simulink model "pid_controller_4inj_dll"  (Simulink 4.00)
settings: Solver=ode5  SolverMode=SingleTasking  StartTime=0.0  StopTime=10  FixedStep=0.0005  RelTol=1e-3
settings Model: Creator=mandic  LastModifiedBy=CAIKA  ExternalInput=[u]  RTWOptions="-aEnforceIntegerDowncast=1 -aExtMode=0 -aFoldNonRolledExpr=1 -aForceParamTrailComments=0 -aGenerateComments=1 -aIgnoreCustomStorageClasses=0 -aIncHierarchyInIds=0 -aInlineInvariantSignals=0 -aLocalBlockOutputs=1 -aLogVarNameModifier=\"rt_\" -aRTWVerbose=1 -aRollThreshold=5 -aShowEliminatedStatements=1"  RTWRetainRTWFile=on  RTWTemplateMakefile=avl_grt_dll_nt.tmf  RTWMakeCommand=make_rtw PROGRAM=pid_controller_4inj  ExtModeTrigMode=oneshot  ExtModeArmWhenConnect=off  ExtModeAutoUpdateStatusClock=off

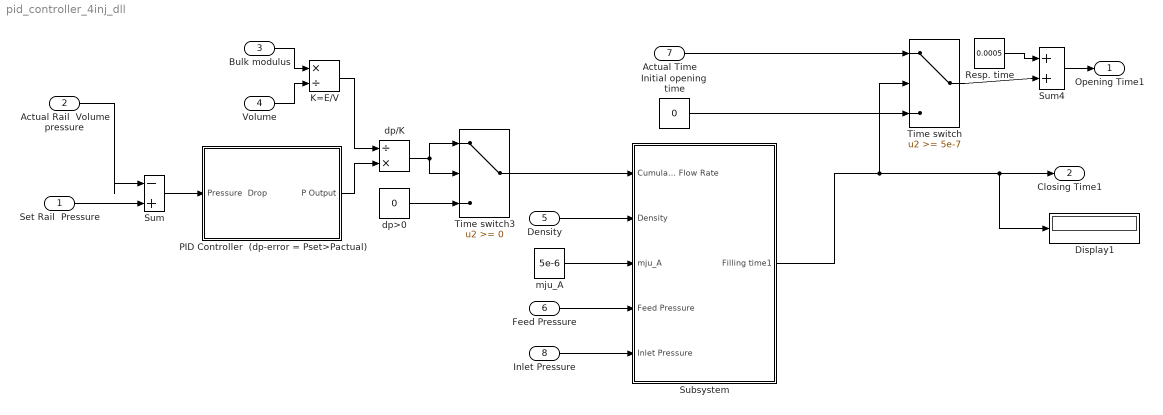
== system pid_controller_4inj_dll ==
  Set Rail  Pressure : Inport  Port=1  LatchInput=off
  Actual Rail  Volume pressure : Inport  Port=2  LatchInput=off
  Bulk modulus : Inport  Port=3  LatchInput=off
  Volume : Inport  Port=4  LatchInput=off
  Density : Inport  Port=5  LatchInput=off
  Feed Pressure : Inport  Port=6  LatchInput=off
  Actual Time : Inport  Port=7  LatchInput=off
  Inlet Pressure : Inport  Port=8  LatchInput=off
  Display1 : Display
      settings: Format=short
  Initial opening  time : Constant  Value=0
  K=E/V : Product  Inputs=*/  Multiplication=Element-wise(.*)  SaturateOnIntegerOverflow=on
  PID Controller  (dp-error = Pset>Pactual) : Subsystem
      settings: RTWFcnNameOpts=Auto  RTWFileNameOpts=Auto
  Resp. time : Constant  Value=0.0005
  Subsystem : Subsystem
      settings: RTWFcnNameOpts=Auto  RTWFileNameOpts=Auto
  Sum : Sum  Inputs=|-+  SaturateOnIntegerOverflow=on
  Sum4 : Sum  Inputs=|++  SaturateOnIntegerOverflow=on
  Time switch : Switch  Threshold=5e-7
  Time switch3 : Switch  Threshold=0
  dp/K : Product  Inputs=/*  Multiplication=Element-wise(.*)  SaturateOnIntegerOverflow=on
  dp>0 : Constant  Value=0
  mju_A : Constant  Value=5e-6
  Opening Time1 : Outport  Port=1
  Closing Time1 : Outport  Port=2
  wires:
  Initial opening  time/1 -> Time switch/3
  Actual Time/1 -> Time switch/1
  Sum/1 -> PID Controller  (dp-error = Pset>Pactual)/1(Pressure  Drop)
  Actual Rail  Volume pressure/1 -> Sum/1
  Set Rail  Pressure/1 -> Sum/2
  Bulk modulus/1 -> K=E/V/1
  Volume/1 -> K=E/V/2
  K=E/V/1 -> dp/K/1
  PID Controller  (dp-error = Pset>Pactual)/1(P Output) -> dp/K/2
  dp/K/1 -> Time switch3/1, Time switch3/2
  Subsystem/1(Filling time1) -> Time switch/2, Closing Time1/1, Display1/1
  Resp. time/1 -> Sum4/1
  Time switch/1 -> Sum4/2
  Sum4/1 -> Opening Time1/1
  dp>0/1 -> Time switch3/3
  Time switch3/1 -> Subsystem/1(Cumulative  Flow Rate)
  Density/1 -> Subsystem/2(Density)
  mju_A/1 -> Subsystem/3(mju_A)
  Feed Pressure/1 -> Subsystem/4(Feed Pressure)
  Inlet Pressure/1 -> Subsystem/5(Inlet Pressure)

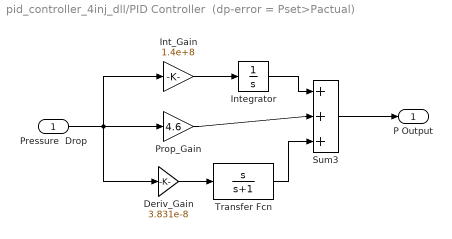
== system pid_controller_4inj_dll/PID Controller  (dp-error = Pset>Pactual) ==
  Pressure  Drop : Inport  Port=1  LatchInput=off
  Deriv_Gain : Gain  Gain=3.831e-8  Multiplication=Element-wise(K.*u)  SaturateOnIntegerOverflow=on
  Int_Gain : Gain  Gain=1.4e+8  Multiplication=Element-wise(K.*u)  SaturateOnIntegerOverflow=on
  Integrator : Integrator  ExternalReset=none  InitialConditionSource=internal  InitialCondition=0  LimitOutput=off  UpperSaturationLimit=inf  LowerSaturationLimit=-inf  ShowSaturationPort=off  ShowStatePort=off  AbsoluteTolerance=auto
  Prop_Gain : Gain  Gain=4.6  Multiplication=Element-wise(K.*u)  SaturateOnIntegerOverflow=on
  Sum3 : Sum  Inputs=|+++  SaturateOnIntegerOverflow=on
  Transfer Fcn : TransferFcn  Numerator=[1 0]  Denominator=[1 1]  AbsoluteTolerance=auto  Realization=auto
  P Output : Outport  Port=1
  wires:
  Int_Gain/1 -> Integrator/1
  Prop_Gain/1 -> Sum3/2
  Integrator/1 -> Sum3/1
  Transfer Fcn/1 -> Sum3/3
  Deriv_Gain/1 -> Transfer Fcn/1
  Pressure  Drop/1 -> Prop_Gain/1, Int_Gain/1, Deriv_Gain/1
  Sum3/1 -> P Output/1

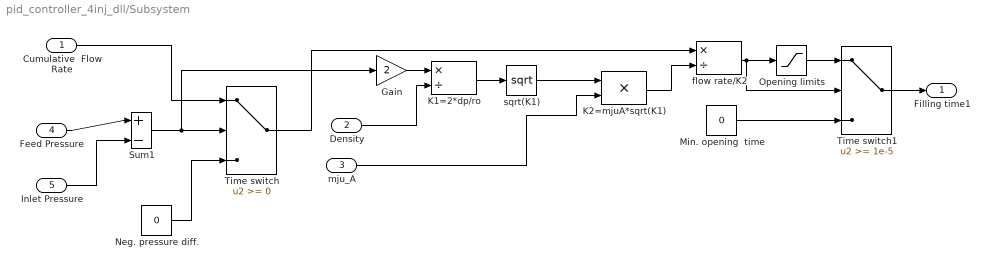
== system pid_controller_4inj_dll/Subsystem ==
  Cumulative  Flow Rate : Inport  Port=1  LatchInput=off
  Density : Inport  Port=2  LatchInput=off
  mju_A : Inport  Port=3  LatchInput=off
  Feed Pressure : Inport  Port=4  LatchInput=off
  Inlet Pressure : Inport  Port=5  LatchInput=off
  Gain : Gain  Gain=2  Multiplication=Element-wise(K.*u)  SaturateOnIntegerOverflow=on
  K1=2*dp/ro : Product  Inputs=*/  Multiplication=Element-wise(.*)  SaturateOnIntegerOverflow=on
  K2=mjuA*sqrt(K1) : Product  Inputs=2  Multiplication=Element-wise(.*)  SaturateOnIntegerOverflow=on
  Min. opening  time : Constant  Value=0
  Neg. pressure diff. : Constant  Value=0
  Opening limits : Saturate  UpperLimit=40e-5  LowerLimit=3e-5  LinearizeAsGain=on
  Sum1 : Sum  Inputs=|+-  SaturateOnIntegerOverflow=on
  Time switch : Switch  Threshold=0
  Time switch1 : Switch  Threshold=1e-5
  flow rate/K2 : Product  Inputs=*/  Multiplication=Element-wise(.*)  SaturateOnIntegerOverflow=on
  sqrt(K1) : Math  Operator=sqrt  OutputSignalType=auto
  Filling time1 : Outport  Port=1
  wires:
  Inlet Pressure/1 -> Sum1/2
  Feed Pressure/1 -> Sum1/1
  Sum1/1 -> Time switch/2, Gain/1
  Neg. pressure diff./1 -> Time switch/3
  Gain/1 -> K1=2*dp/ro/1
  K1=2*dp/ro/1 -> sqrt(K1)/1
  sqrt(K1)/1 -> K2=mjuA*sqrt(K1)/1
  K2=mjuA*sqrt(K1)/1 -> flow rate/K2/2
  flow rate/K2/1 -> Opening limits/1, Time switch1/2
  Opening limits/1 -> Time switch1/1
  Min. opening  time/1 -> Time switch1/3
  Time switch1/1 -> Filling time1/1
  Density/1 -> K1=2*dp/ro/2
  mju_A/1 -> K2=mjuA*sqrt(K1)/2
  Cumulative  Flow Rate/1 -> Time switch/1
  Time switch/1 -> flow rate/K2/1
